simulink model "Full_WaterRunner"  (Simulink 7.9)
settings: Solver=ode45  StartTime=0.0  StopTime=10  MaxStep=1e-2  RelTol=1e-3  AbsTol=1e-3
values from neighbouring files (symbols this model uses):
  frame_inertia = diag([Ix,Iy,Iz])    [SimParam.m]    (also in matlab.mat = [8.0125e-05  0  0; 0  0.000390625  0; 0  0  0.0003145]; simParams.m; simParams_closed.m; speed_cg.mat = [8.0125e-05  0  0; 0  0.000390625  0; 0  0  0.0003145])
  frame_mass = 0.06    [matlab.mat]    (also in simParam.m = 0.03; simParams.m; simParams_closed.m = 0.1; speed_cg.mat)
  L2_inertia = [1.05087286587e-08  0  0; 0  0  0; 0  0  1.05087286587e-08]    [matlab.mat]    (also in simParams.m = diag([I 0 I]); simParams_closed.m = diag([I 0 I]); speed_cg.mat)
  L2_mass = 0.0002653496    [matlab.mat]    (also in simParams.m; simParams_closed.m; speed_cg.mat)
  L3_inertia = [4.24507620885e-07  0  0; 0  0  0; 0  0  4.24507620885e-07]    [matlab.mat]    (also in simParams.m = diag([I 0 I]); simParams_closed.m = diag([I 0 I]); speed_cg.mat)
  L3_mass = 0.0009104656    [matlab.mat]    (also in simParams.m; simParams_closed.m; speed_cg.mat)
  L4_inertia = [1.03972444992e-07  0  0; 0  0  0; 0  0  1.03972444992e-07]    [matlab.mat]    (also in simParams.m = diag([I 0 I]); simParams_closed.m = diag([I 0 I]); speed_cg.mat)
  L4_mass = 0.0005696496    [matlab.mat]    (also in simParams.m; simParams_closed.m; speed_cg.mat)
  motor_inertia = [1.56837175e-06  0  0; 0  1.56837175e-06  0; 0  0  9.00482e-07]    [matlab.mat]    (also in simParams.m = diag([Ix,Iy,Iz]); simParams_closed.m = diag([Ix,Iy,Iz]); speed_cg.mat)
  motor_mass = 0.01    [matlab.mat]    (also in simParam.m; simParams.m; simParams_closed.m; speed_cg.mat)
  water_level = 0    [matlab.mat]    (also in simParam.m; simParams.m = -0.03; simParams_closed.m; speed_cg.mat)
libraries: mblibv1 x61, simulink x4
(part 2 of 2)

== system Full_WaterRunner/motor_FR3/motor_body ==
  Body1 : mblibv1/Bodies/Body  LConnTagsString=CS1  RConnTagsString=CS2  UpdateFromCAD=off  DialogClass=MechanicalBodyBlock  Mass=motor_mass  MassUnits=kg  InertiaUnits=kg*m^2  Inertia=motor_inertia  Shape=Cylinder  ShapeDims=[1 1]  ShapeUnits=m  ShapeUse=false  Density=1  DensityUnits=kg/m^3  DensityUse=false  GraphicsMode=CONVHULL  BodyColorSelMode=COLORPALETTE  BodyColor=[0.87059 0.4902 0]  AttachedToCS=CG  CG=Left$CG$[0 0 0]$CS1$CS1$m$[0 0 0]$Euler X-Y-Z$deg$WORLD$false$none  WorkingFrames=Left$CS1$[0 0 0]$Adjoining$Adjoining$m$[0 0 0]$Euler X-Y-Z$deg$WORLD$true$none#Right$CS2$[0 0 0]$CS1$CS1$m$[0 0 0]$Euler X-Y-Z$deg$WORLD$true$none  CGPos=[0 0 0]  CGRot=[0 0 0]  CS0Pos=[]  CS0Rot=[]  CS1Pos=[0 0 0]  CS1Rot=[0 0 0]  CS2Pos=[0 0 0]  CS2Rot=[0 0 0]  CS3Pos=[]  CS3Rot=[]  CS4Pos=[]  CS4Rot=[]  CS5Pos=[]  CS5Rot=[]  CS6Pos=[]  CS6Rot=[]  CS7Pos=[]  CS7Rot=[]  CS8Pos=[]  CS8Rot=[]  CS9Pos=[]  CS9Rot=[]  CS10Pos=[]  CS10Rot=[]  CS11Pos=[]  CS11Rot=[]  CS12Pos=[]  CS12Rot=[]  CS13Pos=[]  CS13Rot=[]  CS14Pos=[]  CS14Rot=[]  CS15Pos=[]  CS15Rot=[]  CS16Pos=[]  CS16Rot=[]  CS17Pos=[]  CS17Rot=[]  CS18Pos=[]  CS18Rot=[]  CS19Pos=[]  CS19Rot=[]  CS20Pos=[]  CS20Rot=[]
  Weld1 : mblibv1/Joints/Weld  LConnTagsString=__newl0  RConnTagsString=__newr0  UpdateFromCAD=off  NumSAPorts=0  CutJoint=off  MarkAsCut=off  Primitives=weld  PrimitiveProps=W$World$[0 0 0]$weld  DialogClass=JointBlock  WAxis=[0 0 0]
  to_rev : PMIOPort  Port=1  Side=Right
  to_frame : PMIOPort  Port=2  Side=Left
  connections:
  to_frame/RConn1 -- Weld1/LConn1
  to_rev/RConn1 -- Body1/RConn1
  Body1/LConn1 -- Weld1/RConn1
